simulink model "BikeBot_ODE"  (R2021a)
settings: Solver=VariableStepAuto  StartTime=0.0  StopTime=5  RelTol=1e-3
values from neighbouring files (symbols this model uses):
  C_1 = 0    [Bikebot_1.m]
  C_2 = mu*S_T+S_F*cos(lambda)+(I_Txz/w)*cos(lambda)- mu*m_T*z_T    [Bikebot_1.m]
  C_3 = -1*(mu*S_T+S_F*cos(lambda))    [Bikebot_1.m]
  C_4 = (I_Alz/w)*cos(lambda)+mu*(S_A+(I_Tzz/w)*cos(lambda))    [Bikebot_1.m]
  I_All = (m_A*u_A^2) + (I_Axx*(sin(lambda)^2)) + 2*I_Axz*sin(lambda)*cos(lambda) + (I_Azz*(cos(lambda))^2)    [Bikebot_1.m]
  I_Txx = I_Rxx + I_Bxx + I_Hxx + I_Fxx + (m_R*r_R^2) + (m_B*z_B^2) + (m_H*z_H^2) + (m_F*r_F^2)    (= 4.18729508556)    [Bikebot_1.m]
  K0_1 = m_T*z_T    (= -8.82198964)    [Bikebot_1.m]
  K0_2 = -1*S_A    [Bikebot_1.m]
  K0_3 = -1*S_A    [Bikebot_1.m]
  K0_4 = -1*S_A*sin(lambda)    [Bikebot_1.m]
  K2_1 = 0    [Bikebot_1.m]
  K2_2 = ((S_T-m_T*z_T)/w)*cos(lambda)    [Bikebot_1.m]
  K2_3 = 0    [Bikebot_1.m]
  K2_4 = ((S_A+S_F*sin(lambda))/w)*cos(lambda)    [Bikebot_1.m]
  M_1 = I_Txx    (= 4.18729508556)    [Bikebot_1.m]
  M_2 = I_Alx+mu*I_Txz    [Bikebot_1.m]
  M_3 = I_Alx+mu*I_Txz    [Bikebot_1.m]
  M_4 = I_All+2*mu*I_Alz+(mu^2)*I_Tzz    [Bikebot_1.m]
  v = 4    [Bikebot_1.m]
settings Model: Creator=hrish  LastModifiedBy=hrish

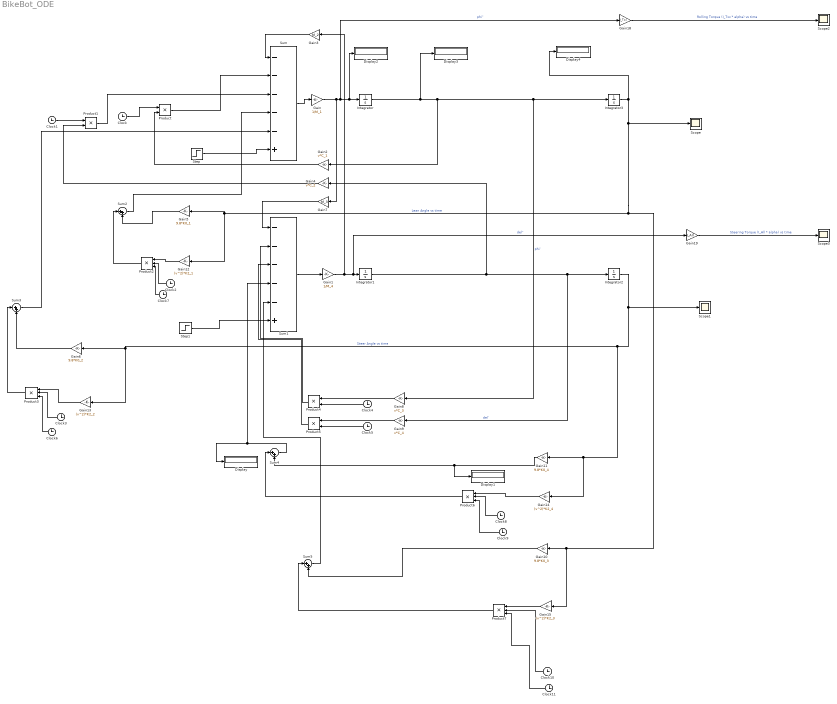
== system BikeBot_ODE ==
  Clock{,1..11} (12 alike) : Clock
  Display{,1..4} (5 alike) : Display
  Gain : Gain  Gain=1/M_1
  Gain1 : Gain  Gain=1/M_4
  Gain10 : Gain  Gain=9.8*K0_3
  Gain11 : Gain  Gain=9.8*K0_4
  Gain12 : Gain  Gain=(v^2)*K2_1
  Gain13 : Gain  Gain=(v^2)*K2_2
  Gain14 : Gain  Gain=(v^2)*K2_4
  Gain15 : Gain  Gain=(v^2)*K2_3
  Gain18 : Gain  Gain=I_Txx
  Gain19 : Gain  Gain=I_All
  Gain2 : Gain  Gain=v*C_1
  Gain3 : Gain  Gain=M_2
  Gain4 : Gain  Gain=v*C_2
  Gain5 : Gain  Gain=9.8*K0_1
  Gain6 : Gain  Gain=9.8*K0_2
  Gain7 : Gain  Gain=M_3
  Gain8 : Gain  Gain=v*C_3
  Gain9 : Gain  Gain=v*C_4
  Integrator{,1..3} (4 alike) : Integrator
  Product{,1,4..5} (4 alike) : Product
  Product{2..3,6..7} (4 alike) : Product  Inputs=3
  Scope{,1..3} (4 alike) : Scope
  Step : Step  SampleTime=0
  Step1 : Step  Time=3  After=50  SampleTime=0
  Sum : Sum  Inputs=-----+
  Sum1 : Sum  Inputs=-----+
  Sum{2..5} (4 alike) : Sum  Inputs=|++
  wires:
  Integrator/1 -> Display3/1, Gain2/1, Gain8/1, Integrator3/1  "phi'"
  Integrator1/1 -> Gain4/1, Gain9/1, Integrator2/1  "del'"
  Gain/1 -> Gain18/1, Display2/1, Integrator/1, Gain7/1  "phi\""
  Gain1/1 -> Gain3/1, Gain19/1, Integrator1/1  "del\""
  Sum1/1 -> Gain1/1
  Sum/1 -> Gain/1
  Gain3/1 -> Sum/1
  Gain4/1 -> Product1/2
  Integrator3/1 -> Scope/1, Gain15/1, Gain10/1, Gain5/1, Gain12/1, Display4/1  "Lean Angle vs time"
  Integrator2/1 -> Scope1/1, Gain14/1, Gain11/1, Gain13/1, Gain6/1  "Steer Angle vs time"
  Gain7/1 -> Sum1/1
  Gain8/1 -> Product4/1
  Gain9/1 -> Product5/1
  Gain10/1 -> Sum5/2
  Gain11/1 -> Display1/1, Sum4/2
  Gain2/1 -> Product/2
  Clock/1 -> Product/1
  Product/1 -> Sum/2
  Clock1/1 -> Product1/1
  Product1/1 -> Sum/3
  Gain12/1 -> Product2/1
  Clock2/1 -> Product2/2
  Product2/1 -> Sum2/1
  Gain5/1 -> Sum2/2
  Sum2/1 -> Sum/4
  Gain13/1 -> Product3/1
  Clock3/1 -> Product3/2
  Product3/1 -> Sum3/1
  Gain6/1 -> Sum3/2
  Sum3/1 -> Sum/5
  Clock4/1 -> Product4/2
  Product4/1 -> Sum1/2
  Clock5/1 -> Product5/2
  Product5/1 -> Sum1/3
  Clock6/1 -> Product3/3
  Clock7/1 -> Product2/3
  Gain14/1 -> Product6/1
  Clock8/1 -> Product6/2
  Clock9/1 -> Product6/3
  Product6/1 -> Sum4/1
  Sum4/1 -> Display/1, Sum1/4
  Clock11/1 -> Product7/3
  Product7/1 -> Sum5/1
  Clock10/1 -> Product7/2
  Gain15/1 -> Product7/1
  Sum5/1 -> Sum1/5
  Gain18/1 -> Scope2/1  "Rolling Torque (I_Txx * alpha) vs time"
  Gain19/1 -> Scope3/1  "Steering Torque (I_All * alpha) vs time"
  Step/1 -> Sum/6
  Step1/1 -> Sum1/6
